simulink model "ben2csys"  (Simulink 6.0)
settings: Solver=ode15s  SolverMode=SingleTasking  StartTime=0.0  StopTime=10  RelTol=1e-3  AbsTol=1e-6
PreLoadFcn:
  | ben2cdat
values from neighbouring files (symbols this model uses):
  a1 = 0.08197    [ben2adat.m]    (also in ben2bdat.m; ben2cdat.m)
  a10 = 0.4078    [ben2adat.m]    (also in ben2bdat.m; ben2cdat.m)
  a11 = 0.3077    [ben2adat.m]    (also in ben2bdat.m; ben2cdat.m)
  a12 = 3.2314    [ben2adat.m]    (also in ben2bdat.m; ben2cdat.m)
  a13 = 0.8597    [ben2adat.m]    (also in ben2bdat.m; ben2cdat.m)
  a14 = -0.002323    [ben2adat.m]    (also in ben2bdat.m; ben2cdat.m)
  a15 = -0.01139    [ben2adat.m]    (also in ben2bdat.m; ben2cdat.m)
  a16 = 45.112    [ben2adat.m]    (also in ben2bdat.m; ben2cdat.m)
  a2 = 0.02296    [ben2adat.m]    (also in ben2bdat.m; ben2cdat.m)
  a3 = -0.004879    [ben2adat.m]    (also in ben2bdat.m; ben2cdat.m)
  a4 = -0.03402    [ben2adat.m]    (also in ben2bdat.m; ben2cdat.m)
  a5 = 0.2551    [ben2adat.m]    (also in ben2bdat.m; ben2cdat.m)
  a6 = 0.02549    [ben2adat.m]    (also in ben2bdat.m; ben2cdat.m)
  a7 = -0.1199    [ben2adat.m]    (also in ben2bdat.m; ben2cdat.m)
  a8 = -0.4283    [ben2adat.m]    (also in ben2bdat.m; ben2cdat.m)
  a9 = 0.6645    [ben2adat.m]    (also in ben2bdat.m; ben2cdat.m)
  b1 = 0.007429    [ben2adat.m]    (also in ben2bdat.m; ben2cdat.m)
  b10 = -0.1037    [ben2adat.m]    (also in ben2bdat.m; ben2cdat.m)
  b11 = 0.3077    [ben2adat.m]    (also in ben2bdat.m; ben2cdat.m)
  b12 = 3.2314    [ben2adat.m]    (also in ben2bdat.m; ben2cdat.m)
  b13 = 0    [ben2adat.m]    (also in ben2bdat.m; ben2cdat.m)
  b14 = 0.002115    [ben2adat.m]    (also in ben2bdat.m; ben2cdat.m)
  b15 = -0.01139    [ben2adat.m]    (also in ben2bdat.m; ben2cdat.m)
  b16 = 45.112    [ben2adat.m]    (also in ben2bdat.m; ben2cdat.m)
  b17 = 0.4040    (= 0.404)    [ben2adat.m]    (also in ben2bdat.m; ben2cdat.m)
  b2 = 0.0752    [ben2adat.m]    (also in ben2bdat.m; ben2cdat.m)
  b3 = 0.06919    [ben2adat.m]    (also in ben2bdat.m; ben2cdat.m)
  b4 = -0.8272    [ben2adat.m]    (also in ben2bdat.m; ben2cdat.m)
  b5 = 0.03861    [ben2adat.m]    (also in ben2bdat.m; ben2cdat.m)
  b6 = -0.3616    [ben2adat.m]    (also in ben2bdat.m; ben2cdat.m)
  b7 = -0.3930    (= -0.393)    [ben2adat.m]    (also in ben2bdat.m; ben2cdat.m)
  b8 = -0.03882    [ben2adat.m]    (also in ben2bdat.m; ben2cdat.m)
  b9 = 0.8064    [ben2adat.m]    (also in ben2bdat.m; ben2cdat.m)
  c1 = -0.01523    [ben2adat.m]    (also in ben2bdat.m; ben2cdat.m)
  c2 = 0.06768    [ben2adat.m]    (also in ben2bdat.m; ben2cdat.m)
  c3 = 0.01514    [ben2adat.m]    (also in ben2bdat.m; ben2cdat.m)
  c4 = 0.002194    [ben2adat.m]    (also in ben2bdat.m; ben2cdat.m)
  c5 = 0.07528    [ben2adat.m]    (also in ben2bdat.m; ben2cdat.m)
  c6 = 0.0002996    [ben2adat.m]    (also in ben2bdat.m = -0.0002996; ben2cdat.m = -0.0002996)
  c7 = 3030.76    [ben2adat.m]    (also in ben2bdat.m; ben2cdat.m)
  gd1 = 1    [ben2adat.m]    (also in ben2bdat.m; ben2cdat.m = [1/950,1]; ben3adat.m = [1,6,13]; ben3bdat.m = [1,6,13])
  gd10 = [1/28,1.4536,1]    [ben2adat.m]    (also in ben2bdat.m; ben2cdat.m)
  gd11 = k13    (= 2.9)    [ben2adat.m]    (also in ben2bdat.m; ben2cdat.m)
  gd12 = [1/325/325,0.5/325,1]    [ben2adat.m]    (also in ben2bdat.m; ben2cdat.m; ben3bdat.m = [1,0])
  gd131 = [1/665/665,.8/665,1]    [ben2cdat.m]    (also in ben3bdat.m = [T2,0])
  gd132 = [1/260/260,0.5/260,1]    [ben2cdat.m]    (also in ben3bdat.m = [1,-1.785,.9988])
  gd13d = [1/2500,1]    [ben2cdat.m]
  gd14 = 1    [ben2adat.m]    (also in ben2bdat.m; ben2cdat.m)
  gd15 = [1,0]    [ben2adat.m]    (also in ben2bdat.m; ben2cdat.m)
  gd161 = [1/70,1]    [ben2bdat.m]    (also in ben2cdat.m)
  gd162 = [1/165/165,1/165,1]    [ben2bdat.m]    (also in ben2cdat.m)
  gd163 = [1/725/725,.8/725,1]    [ben2cdat.m]
  gd17 = [1,0]    [ben2adat.m]    (also in ben2bdat.m; ben2cdat.m)
  gd2 = [1/220,1]    [ben2adat.m]    (also in ben2bdat.m; ben2cdat.m; ben3adat.m = [1,6,13]; ben3bdat.m = [1,6,13])
  gd3 = [1/85/85,1.2/85,1]    [ben2adat.m]    (also in ben2bdat.m; ben2cdat.m; ben3adat.m = [1,-1]; ben3bdat.m = [1,-1])
  gd4 = 1    [ben2adat.m]    (also in ben2bdat.m; ben2cdat.m = [1/775/775,1/775,1]; ben3adat.m = [1,-0.6667]; ben3bdat.m = [1,-0.6667])
  gd5 = [1/170,1]    [ben2adat.m]    (also in ben2bdat.m; ben2cdat.m; ben3adat.m = [1,-1]; ben3bdat.m = [1,-1])
  gd61 = [1/80,1]    [ben2adat.m]    (also in ben2bdat.m; ben2cdat.m)
  gd62 = [1/160/160,0.6/160,1]    [ben2adat.m]    (also in ben2bdat.m; ben2cdat.m)
  gd63 = [1/1600,1]    [ben2adat.m]    (also in ben2bdat.m; ben2cdat.m)
  gd64 = [1/250/250,.6/250,1]    [ben2cdat.m]
  gd65 = [1/300/300,.6/300,1]    [ben2cdat.m]
  gd66 = [1/575/575,.8/575,1]    [ben2cdat.m]
  gd67 = [1/500/500,.6/500,1]    [ben2cdat.m]
  gd7 = [1,0]    [ben2adat.m]    (also in ben2bdat.m; ben2cdat.m; ben3adat.m = [1,-0.9277]; ben3bdat.m = [1,-0.9277])
  gd8 = 1    [ben2adat.m]    (also in ben2bdat.m; ben2cdat.m = [1/526.3,1])
  gd91 = [1,0]    [ben2adat.m]    (also in ben2bdat.m; ben2cdat.m; ben3bdat.m = [1,.25*200,200*200])
  gd92 = [1/50,1]    [ben2adat.m]    (also in ben2bdat.m; ben2cdat.m; ben3bdat.m = [1,0])
  gn1 = 1    [ben2adat.m]    (also in ben2bdat.m; ben2cdat.m; ben3adat.m = -15*[1,1.5]; ben3bdat.m = -15*[1,1.5])
  gn10 = [-1,0]    [ben2adat.m]    (also in ben2bdat.m; ben2cdat.m)
  gn11 = k14    (= 0.66)    [ben2adat.m]    (also in ben2bdat.m; ben2cdat.m)
  gn12 = [1,0]    [ben2adat.m]    (also in ben2bdat.m; ben2cdat.m; ben3bdat.m = 1)
  gn131 = [1/665/665,.08/665,1]    [ben2cdat.m]    (also in ben3bdat.m = [1,-1])
  gn132 = [1/800/800,.12/800,1]    [ben2cdat.m]    (also in ben3bdat.m = .9994*[1,-1.786,1])
  gn13d = [0.4/130,0.4]    [ben2cdat.m]
  gn14 = 0.2 * k14    (= 0.132)    [ben2adat.m]    (also in ben2bdat.m; ben2cdat.m)
  gn15 = [1/30,1]    [ben2adat.m]    (also in ben2bdat.m; ben2cdat.m)
  gn161 = [1/45,1]    [ben2bdat.m]    (also in ben2cdat.m)
  gn162 = 1    [ben2bdat.m]    (also in ben2cdat.m)
  gn163 = [1/725/725,.08/725,1]    [ben2cdat.m]
  gn17 = k12    (= 0.565)    [ben2adat.m]    (also in ben2bdat.m; ben2cdat.m)
  gn2 = 1    [ben2adat.m]    (also in ben2bdat.m; ben2cdat.m; ben3adat.m = [-0.1,9]; ben3bdat.m = [-0.1,9])
  gn3 = 1    [ben2adat.m]    (also in ben2bdat.m; ben2cdat.m; ben3adat.m = .2625*[1,-0.9048]; ben3bdat.m = .2625*[1,-0.9048])
  gn4 = 1    [ben2adat.m]    (also in ben2bdat.m; ben2cdat.m; ben3adat.m = 1.7*[1,-0.9608]; ben3bdat.m = 1.7*[1,-0.9608])
  gn5 = 1    [ben2adat.m]    (also in ben2bdat.m; ben2cdat.m; ben3adat.m = 1.035*[1,-0.9324]; ben3bdat.m = 1.035*[1,-0.9324])
  gn61 = [1,0]    [ben2adat.m]    (also in ben2bdat.m; ben2cdat.m)
  gn62 = [1/30,1]    [ben2adat.m]    (also in ben2bdat.m; ben2cdat.m)
  gn63 = 1    [ben2adat.m]    (also in ben2bdat.m; ben2cdat.m)
  gn64 = [1/250/250,.06/250,1]    [ben2cdat.m]
  gn65 = [1/350/350,.06/350,1]    [ben2cdat.m]
  gn66 = [1/660/660,.4/660,1]    [ben2cdat.m]
  gn67 = [1/850/850,.06/850,1]    [ben2cdat.m]
  gn7 = 1    [ben2adat.m]    (also in ben2bdat.m; ben2cdat.m; ben3adat.m = 0.0362*[1,1]; ben3bdat.m = 0.0362*[1,1])
  gn8 = 1    [ben2adat.m]    (also in ben2bdat.m; ben2cdat.m = [(-1)/526.1,1])
  gn91 = [1,1.5]    [ben2adat.m]    (also in ben2bdat.m; ben2cdat.m; ben3bdat.m = 40000)
  gn92 = [1/150,1]    [ben2adat.m]    (also in ben2bdat.m; ben2cdat.m; ben3bdat.m = 1)
  k1 = 1    [ben2adat.m]    (also in ben2bdat.m; ben2cdat.m)
  k10 = 0    [ben2adat.m]    (also in ben2bdat.m; ben2cdat.m = 0.2)
  k11 = 0.0112    [ben2adat.m]    (also in ben2bdat.m; ben2cdat.m)
  k2 = 1.25    [ben2adat.m]    (also in ben2bdat.m; ben2cdat.m)
  k3 = 0.001244    [ben2adat.m]    (also in ben2bdat.m; ben2cdat.m)
  k4 = 0.1    [ben2adat.m]    (also in ben2bdat.m; ben2cdat.m)
  k5 = 0.01125    [ben2adat.m]    (also in ben2bdat.m; ben2cdat.m)
  k6 = 0.06    [ben2adat.m]    (also in ben2bdat.m; ben2cdat.m)
  k7 = 0    [ben2adat.m]    (also in ben2bdat.m; ben2cdat.m = 0.5)
  k8 = 0    [ben2adat.m]    (also in ben2bdat.m; ben2cdat.m = 0.2)
  k9 = 29.82    [ben2adat.m]    (also in ben2bdat.m; ben2cdat.m)
settings Model: Creator=The MathWorks Inc.  LastModifiedBy=batserve  ExtModeTrigMode=oneshot  ExtModeArmWhenConnect=off  ExtModeAutoUpdateStatusClock=off
settings DataIOCC: ExternalInput=[]  InitialState=[]  LimitDataPoints=off  SaveOutput=off  SaveTime=off
settings OptimizationCC: BooleanDataType=off
settings DebuggingCC: CheckExecutionContextPreStartOutputMsg=on  CheckExecutionContextRuntimeOutputMsg=on  SolverPrmCheckMsg=none  IntegerOverflowMsg=none
settings HardwareCC: TargetUnknown=on

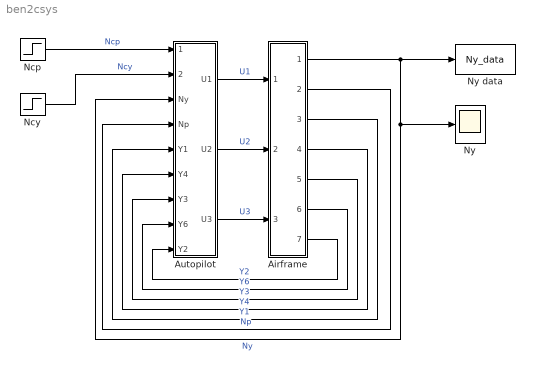
== system ben2csys ==
  Airframe : Subsystem  PropExecContextAcrossSSBoundary=on
  Autopilot : Subsystem  PropExecContextAcrossSSBoundary=on
  Ncp : Step  Time=0  After=0  SampleTime=0
  Ncy : Step  Time=0  SampleTime=0
  Ny : Scope
      settings: TickLabels=on  TimeRange=10  YMin=-0.2  YMax=1.6  DataFormat=Array
  Ny data : ToWorkspace  VariableName=Ny_data  SampleTime=-1  SaveFormat=Array
  wires:
  Airframe/7(Y2) -> Autopilot/9(Y2)  "Y2"
  Airframe/6(Y6) -> Autopilot/8(Y6)  "Y6"
  Airframe/5(Y3) -> Autopilot/7(Y3)  "Y3"
  Airframe/4(Y4) -> Autopilot/6(Y4)  "Y4"
  Airframe/3(Y1) -> Autopilot/5(Y1)  "Y1"
  Airframe/2(Np) -> Autopilot/4(Np)  "Np"
  Ncp/1 -> Autopilot/1(Ncp)  "Ncp"
  Autopilot/1(U1) -> Airframe/1(U1)  "U1"
  Autopilot/2(U2) -> Airframe/2(U2)  "U2"
  Autopilot/3(U3) -> Airframe/3(U3)  "U3"
  Ncy/1 -> Autopilot/2(Ncy)  "Ncy"
  Airframe/1(Ny) -> Ny/1, Autopilot/3(Ny), Ny data/1  "Ny"

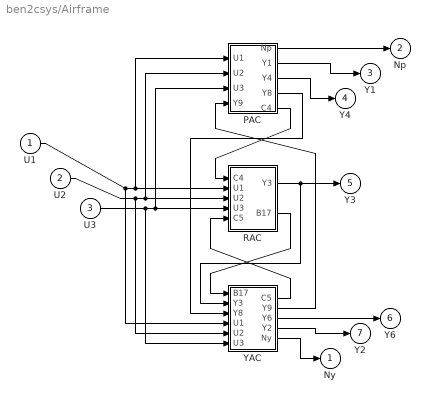
== system ben2csys/Airframe ==
  U1 : Inport  Port=1  LatchInput=off
  U2 : Inport  Port=2  LatchInput=off
  U3 : Inport  Port=3  LatchInput=off
  PAC : Subsystem  PropExecContextAcrossSSBoundary=on
  RAC : Subsystem  PropExecContextAcrossSSBoundary=on
  YAC : Subsystem  PropExecContextAcrossSSBoundary=on
  Ny : Outport  InitialOutput=0
  Np : Outport  Port=2  InitialOutput=0
  Y1 : Outport  Port=3  InitialOutput=0
  Y4 : Outport  Port=4  InitialOutput=0
  Y3 : Outport  Port=5  InitialOutput=0
  Y6 : Outport  Port=6  InitialOutput=0
  Y2 : Outport  Port=7  InitialOutput=0
  wires:
  PAC/5(C4) -> RAC/1(C4)
  PAC/1(Np) -> Np/1
  PAC/2(Y1) -> Y1/1
  PAC/3(Y4) -> Y4/1
  RAC/2(B17) -> YAC/1(B17)
  YAC/5(Ny) -> Ny/1
  YAC/4(Y2) -> Y2/1
  YAC/3(Y6) -> Y6/1
  YAC/2(Y9) -> PAC/4(Y9)
  PAC/4(Y8) -> YAC/3(Y8)
  YAC/1(C5) -> RAC/5(C5)
  RAC/1(Y3) -> Y3/1, YAC/2(Y3)
  U1/1 -> YAC/4(U1), RAC/2(U1), PAC/1(U1)
  U2/1 -> YAC/5(U2), RAC/3(U2), PAC/2(U2)
  U3/1 -> YAC/6(U3), RAC/4(U3), PAC/3(U3)

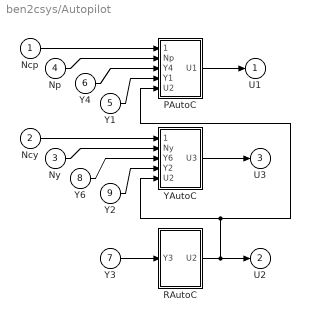
== system ben2csys/Autopilot ==
  Ncp : Inport  Port=1  LatchInput=off
  Ncy : Inport  Port=2  LatchInput=off
  Ny : Inport  Port=3  LatchInput=off
  Np : Inport  Port=4  LatchInput=off
  Y1 : Inport  Port=5  LatchInput=off
  Y4 : Inport  Port=6  LatchInput=off
  Y3 : Inport  Port=7  LatchInput=off
  Y6 : Inport  Port=8  LatchInput=off
  Y2 : Inport  Port=9  LatchInput=off
  PAutoC : Subsystem  PropExecContextAcrossSSBoundary=on
  RAutoC : Subsystem  PropExecContextAcrossSSBoundary=on
  YAutoC : Subsystem  PropExecContextAcrossSSBoundary=on
  U1 : Outport  InitialOutput=0
  U2 : Outport  Port=2  InitialOutput=0
  U3 : Outport  Port=3  InitialOutput=0
  wires:
  RAutoC/1(U2) -> U2/1, YAutoC/5(U2), PAutoC/5(U2)
  Y3/1 -> RAutoC/1(Y3)
  Y2/1 -> YAutoC/4(Y2)
  YAutoC/1(U3) -> U3/1
  Y6/1 -> YAutoC/3(Y6)
  Ny/1 -> YAutoC/2(Ny)
  Ncy/1 -> YAutoC/1(Ncy)
  Y1/1 -> PAutoC/4(Y1)
  PAutoC/1(U1) -> U1/1
  Y4/1 -> PAutoC/3(Y4)
  Np/1 -> PAutoC/2(Np)
  Ncp/1 -> PAutoC/1(Ncp)

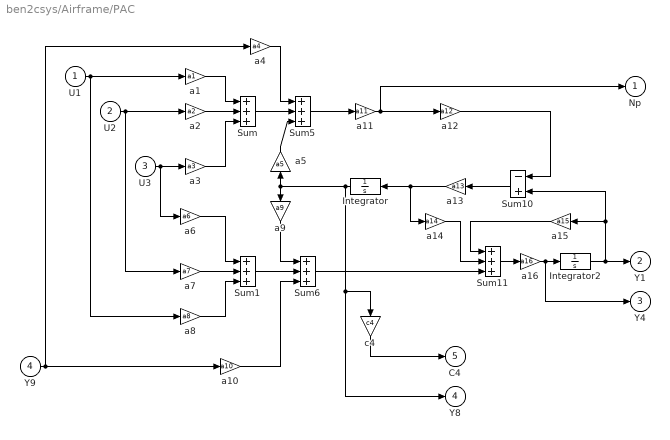
== system ben2csys/Airframe/PAC ==
  U1 : Inport  Port=1  LatchInput=off
  U2 : Inport  Port=2  LatchInput=off
  U3 : Inport  Port=3  LatchInput=off
  Y9 : Inport  Port=4  LatchInput=off
  Integrator : Integrator  Orientation=left
  Integrator2 : Integrator
  Sum{,1,5..6,11} (5 alike) : Sum  Inputs=3  SaturateOnIntegerOverflow=on  InputSameDT=on
  Sum10 : Sum  Orientation=left  Inputs=-+  SaturateOnIntegerOverflow=on  InputSameDT=on
  a1 : Gain  Gain=a1  SaturateOnIntegerOverflow=on
  a10 : Gain  Gain=a10  SaturateOnIntegerOverflow=on
  a11 : Gain  Gain=a11  SaturateOnIntegerOverflow=on
  a12 : Gain  Gain=a12  SaturateOnIntegerOverflow=on
  a13 : Gain  Orientation=left  Gain=a13  SaturateOnIntegerOverflow=on
  a14 : Gain  Gain=a14  SaturateOnIntegerOverflow=on
  a15 : Gain  Orientation=left  Gain=a15  SaturateOnIntegerOverflow=on
  a16 : Gain  Gain=a16  SaturateOnIntegerOverflow=on
  a2 : Gain  Gain=a2  SaturateOnIntegerOverflow=on
  a3 : Gain  Gain=a3  SaturateOnIntegerOverflow=on
  a4 : Gain  Gain=a4  SaturateOnIntegerOverflow=on
  a5 : Gain  Orientation=up  Gain=a5  SaturateOnIntegerOverflow=on
  a6 : Gain  Gain=a6  SaturateOnIntegerOverflow=on
  a7 : Gain  Gain=a7  SaturateOnIntegerOverflow=on
  a8 : Gain  Gain=a8  SaturateOnIntegerOverflow=on
  a9 : Gain  Orientation=down  Gain=a9  SaturateOnIntegerOverflow=on
  c4 : Gain  Orientation=down  Gain=c4  SaturateOnIntegerOverflow=on
  Np : Outport  InitialOutput=0
  Y1 : Outport  Port=2  InitialOutput=0
  Y4 : Outport  Port=3  InitialOutput=0
  Y8 : Outport  Port=4  InitialOutput=0
  C4 : Outport  Port=5  InitialOutput=0
  wires:
  a1/1 -> Sum/1
  a3/1 -> Sum/3
  a8/1 -> Sum1/3
  a6/1 -> Sum1/1
  Integrator2/1 -> Sum10/2, a15/1, Y1/1
  a13/1 -> a14/1, Integrator/1
  Sum/1 -> Sum5/2
  a5/1 -> Sum5/3
  a4/1 -> Sum5/1
  Sum5/1 -> a11/1
  a11/1 -> Np/1, a12/1
  a12/1 -> Sum10/1
  Sum10/1 -> a13/1
  Sum6/1 -> Sum11/3
  a14/1 -> Sum11/2
  a15/1 -> Sum11/1
  Sum11/1 -> a16/1
  a10/1 -> Sum6/3
  Sum1/1 -> Sum6/2
  a9/1 -> Sum6/1
  a16/1 -> Y4/1, Integrator2/1
  U3/1 -> a6/1, a3/1
  a7/1 -> Sum1/2
  a2/1 -> Sum/2
  U1/1 -> a8/1, a1/1
  U2/1 -> a7/1, a2/1
  Y9/1 -> a10/1, a4/1
  Integrator/1 -> c4/1, Y8/1, a9/1, a5/1
  c4/1 -> C4/1

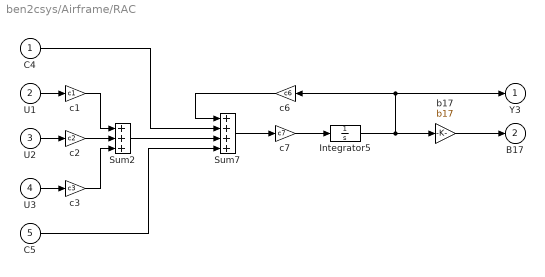
== system ben2csys/Airframe/RAC ==
  C4 : Inport  Port=1  LatchInput=off
  U1 : Inport  Port=2  LatchInput=off
  U2 : Inport  Port=3  LatchInput=off
  U3 : Inport  Port=4  LatchInput=off
  C5 : Inport  Port=5  LatchInput=off
  Integrator5 : Integrator
  Sum2 : Sum  Inputs=3  SaturateOnIntegerOverflow=on  InputSameDT=on
  Sum7 : Sum  Inputs=4  SaturateOnIntegerOverflow=on  InputSameDT=on
  b17 : Gain  Gain=b17  SaturateOnIntegerOverflow=on
  c1 : Gain  Gain=c1  SaturateOnIntegerOverflow=on
  c2 : Gain  Gain=c2  SaturateOnIntegerOverflow=on
  c3 : Gain  Gain=c3  SaturateOnIntegerOverflow=on
  c6 : Gain  Orientation=left  Gain=c6  SaturateOnIntegerOverflow=on
  c7 : Gain  Gain=c7  SaturateOnIntegerOverflow=on
  Y3 : Outport  InitialOutput=0
  B17 : Outport  Port=2  InitialOutput=0
  wires:
  Integrator5/1 -> Y3/1, c6/1, b17/1
  b17/1 -> B17/1
  c6/1 -> Sum7/1
  c7/1 -> Integrator5/1
  Sum7/1 -> c7/1
  C5/1 -> Sum7/4
  C4/1 -> Sum7/2
  Sum2/1 -> Sum7/3
  U3/1 -> c3/1
  c3/1 -> Sum2/3
  c1/1 -> Sum2/1
  U1/1 -> c1/1
  c2/1 -> Sum2/2
  U2/1 -> c2/1

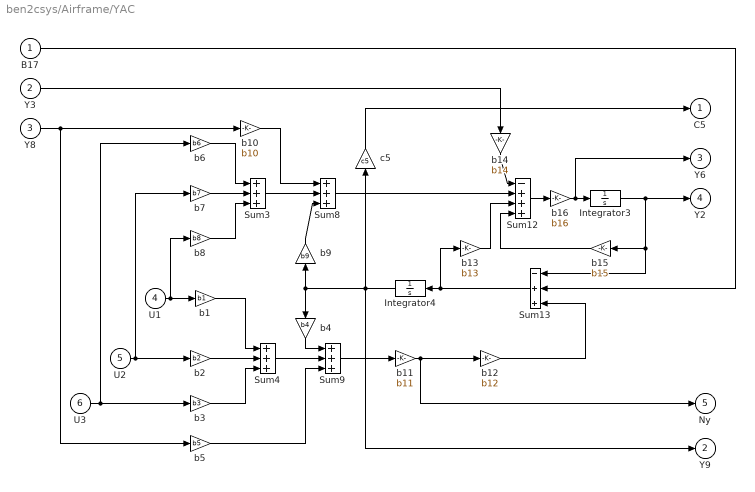
== system ben2csys/Airframe/YAC ==
  B17 : Inport  Port=1  LatchInput=off
  Y3 : Inport  Port=2  LatchInput=off
  Y8 : Inport  Port=3  LatchInput=off
  U1 : Inport  Port=4  LatchInput=off
  U2 : Inport  Port=5  LatchInput=off
  U3 : Inport  Port=6  LatchInput=off
  Integrator3 : Integrator
  Integrator4 : Integrator  Orientation=left
  Sum12 : Sum  Inputs=-+++  SaturateOnIntegerOverflow=on  InputSameDT=on
  Sum13 : Sum  Orientation=left  Inputs=-++  SaturateOnIntegerOverflow=on  InputSameDT=on
  Sum{3..4,8..9} (4 alike) : Sum  Inputs=3  SaturateOnIntegerOverflow=on  InputSameDT=on
  b1 : Gain  Gain=b1  SaturateOnIntegerOverflow=on
  b10 : Gain  Gain=b10  SaturateOnIntegerOverflow=on
  b11 : Gain  Gain=b11  SaturateOnIntegerOverflow=on
  b12 : Gain  Gain=b12  SaturateOnIntegerOverflow=on
  b13 : Gain  Gain=b13  SaturateOnIntegerOverflow=on
  b14 : Gain  Orientation=down  Gain=b14  SaturateOnIntegerOverflow=on
  b15 : Gain  Orientation=left  Gain=b15  SaturateOnIntegerOverflow=on
  b16 : Gain  Gain=b16  SaturateOnIntegerOverflow=on
  b2 : Gain  Gain=b2  SaturateOnIntegerOverflow=on
  b3 : Gain  Gain=b3  SaturateOnIntegerOverflow=on
  b4 : Gain  Orientation=down  Gain=b4  SaturateOnIntegerOverflow=on
  b5 : Gain  Gain=b5  SaturateOnIntegerOverflow=on
  b6 : Gain  Gain=b6  SaturateOnIntegerOverflow=on
  b7 : Gain  Gain=b7  SaturateOnIntegerOverflow=on
  b8 : Gain  Gain=b8  SaturateOnIntegerOverflow=on
  b9 : Gain  Orientation=up  Gain=b9  SaturateOnIntegerOverflow=on
  c5 : Gain  Orientation=up  Gain=c5  SaturateOnIntegerOverflow=on
  C5 : Outport  InitialOutput=0
  Y9 : Outport  Port=2  InitialOutput=0
  Y6 : Outport  Port=3  InitialOutput=0
  Y2 : Outport  Port=4  InitialOutput=0
  Ny : Outport  Port=5  InitialOutput=0
  wires:
  Integrator3/1 -> Sum13/1, b15/1, Y2/1
  Y3/1 -> b14/1
  b6/1 -> Sum3/1
  b8/1 -> Sum3/3
  Y8/1 -> b5/1, b10/1
  b3/1 -> Sum4/3
  b1/1 -> Sum4/1
  Sum13/1 -> b13/1, Integrator4/1
  c5/1 -> C5/1
  U3/1 -> b6/1, b3/1
  U2/1 -> b7/1, b2/1
  U1/1 -> b8/1, b1/1
  b16/1 -> Y6/1, Integrator3/1
  Sum9/1 -> b11/1
  b11/1 -> Ny/1, b12/1
  Sum8/1 -> Sum12/2
  b5/1 -> Sum9/3
  b4/1 -> Sum9/1
  b9/1 -> Sum8/3
  b2/1 -> Sum4/2
  b13/1 -> Sum12/3
  b15/1 -> Sum12/4
  b10/1 -> Sum8/1
  Sum3/1 -> Sum8/2
  b7/1 -> Sum3/2
  b14/1 -> Sum12/1
  Sum12/1 -> b16/1
  b12/1 -> Sum13/3
  Sum4/1 -> Sum9/2
  Integrator4/1 -> b4/1, b9/1, Y9/1, c5/1
  B17/1 -> Sum13/2

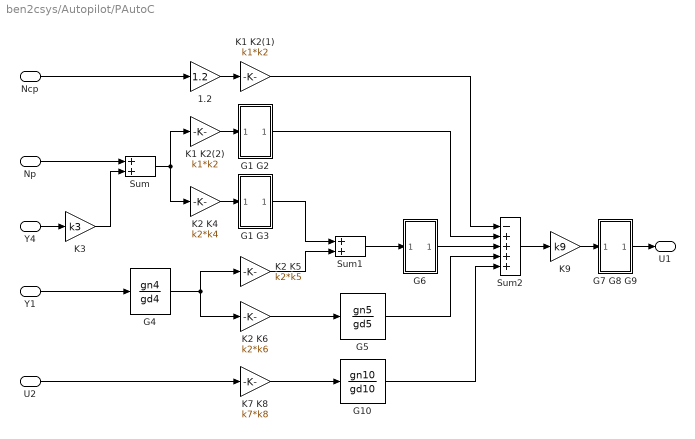
== system ben2csys/Autopilot/PAutoC ==
  Ncp : Inport  Port=1  LatchInput=off
  Np : Inport  Port=2  LatchInput=off
  Y4 : Inport  Port=3  LatchInput=off
  Y1 : Inport  Port=4  LatchInput=off
  U2 : Inport  Port=5  LatchInput=off
  1.2 : Gain  Gain=1.2  SaturateOnIntegerOverflow=on
  G1 G2 : Subsystem  PropExecContextAcrossSSBoundary=on
  G1 G3 : Subsystem  PropExecContextAcrossSSBoundary=on
  G10 : TransferFcn  Numerator=gn10  Denominator=gd10
  G4 : TransferFcn  Numerator=gn4  Denominator=gd4
  G5 : TransferFcn  Numerator=gn5  Denominator=gd5
  G6 : Subsystem  PropExecContextAcrossSSBoundary=on
  G7 G8 G9 : Subsystem  PropExecContextAcrossSSBoundary=on
  K1 K2(1) : Gain  Gain=k1*k2  SaturateOnIntegerOverflow=on
  K1 K2(2) : Gain  Gain=k1*k2  SaturateOnIntegerOverflow=on
  K2 K4 : Gain  Gain=k2*k4  SaturateOnIntegerOverflow=on
  K2 K5 : Gain  Gain=k2*k5  SaturateOnIntegerOverflow=on
  K2 K6 : Gain  Gain=k2*k6  SaturateOnIntegerOverflow=on
  K3 : Gain  Gain=k3  SaturateOnIntegerOverflow=on
  K7 K8 : Gain  Gain=k7*k8  SaturateOnIntegerOverflow=on
  K9 : Gain  Gain=k9  SaturateOnIntegerOverflow=on
  Sum : Sum  Inputs=2  SaturateOnIntegerOverflow=on  InputSameDT=on
  Sum1 : Sum  Inputs=2  SaturateOnIntegerOverflow=on  InputSameDT=on
  Sum2 : Sum  Inputs=-++++  SaturateOnIntegerOverflow=on  InputSameDT=on
  U1 : Outport  InitialOutput=0
  wires:
  G7 G8 G9/1(Out) -> U1/1
  K9/1 -> G7 G8 G9/1(In)
  Y1/1 -> G4/1
  Y4/1 -> K3/1
  Np/1 -> Sum/1
  Ncp/1 -> 1.2/1
  Sum2/1 -> K9/1
  G1 G3/1(Out) -> Sum1/1
  K2 K4/1 -> G1 G3/1(In)
  Sum/1 -> K1 K2(2)/1, K2 K4/1
  K1 K2(2)/1 -> G1 G2/1(In)
  G1 G2/1(Out) -> Sum2/2
  K1 K2(1)/1 -> Sum2/1
  K3/1 -> Sum/2
  G6/1(Out) -> Sum2/3
  Sum1/1 -> G6/1(In)
  G5/1 -> Sum2/4
  K2 K5/1 -> Sum1/2
  1.2/1 -> K1 K2(1)/1
  G4/1 -> K2 K6/1, K2 K5/1
  K2 K6/1 -> G5/1
  U2/1 -> K7 K8/1
  K7 K8/1 -> G10/1
  G10/1 -> Sum2/5

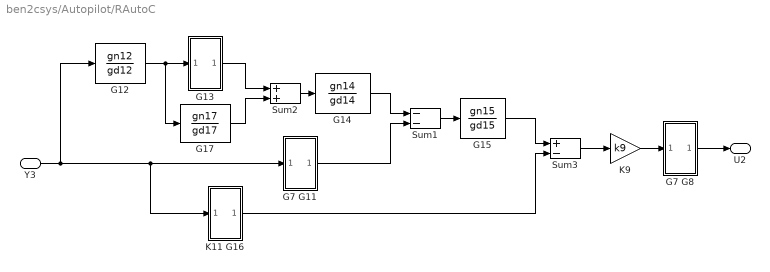
== system ben2csys/Autopilot/RAutoC ==
  Y3 : Inport  Port=1  LatchInput=off
  G12 : TransferFcn  Numerator=gn12  Denominator=gd12
  G13 : Subsystem  PropExecContextAcrossSSBoundary=on
  G14 : TransferFcn  Numerator=gn14  Denominator=gd14
  G15 : TransferFcn  Numerator=gn15  Denominator=gd15
  G17 : TransferFcn  Numerator=gn17  Denominator=gd17
  G7 G11 : Subsystem  PropExecContextAcrossSSBoundary=on
  G7 G8 : Subsystem  PropExecContextAcrossSSBoundary=on
  K11 G16 : Subsystem  PropExecContextAcrossSSBoundary=on
  K9 : Gain  Gain=k9  SaturateOnIntegerOverflow=on
  Sum1 : Sum  Inputs=--  SaturateOnIntegerOverflow=on  InputSameDT=on
  Sum2 : Sum  Inputs=2  SaturateOnIntegerOverflow=on  InputSameDT=on
  Sum3 : Sum  Inputs=+-  SaturateOnIntegerOverflow=on  InputSameDT=on
  U2 : Outport  InitialOutput=0
  wires:
  K11 G16/1(Out) -> Sum3/2
  G15/1 -> Sum3/1
  G7 G11/1(Out) -> Sum1/2
  G12/1 -> G17/1, G13/1(In)
  Sum3/1 -> K9/1
  Sum1/1 -> G15/1
  G14/1 -> Sum1/1
  Sum2/1 -> G14/1
  G13/1(Out) -> Sum2/1
  G17/1 -> Sum2/2
  Y3/1 -> G7 G11/1(In), K11 G16/1(In), G12/1
  G7 G8/1(Out) -> U2/1
  K9/1 -> G7 G8/1(In)

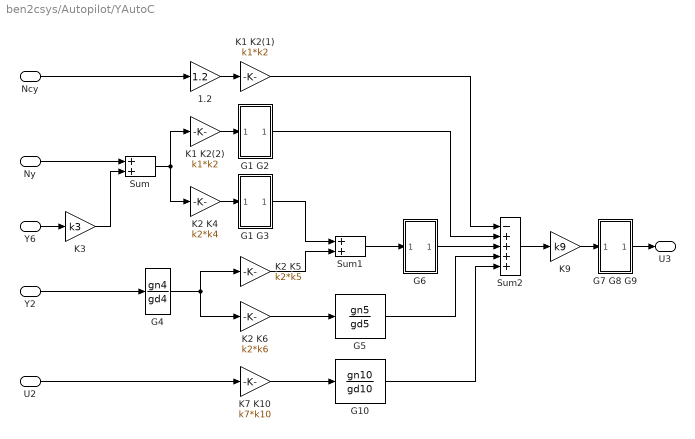
== system ben2csys/Autopilot/YAutoC ==
  Ncy : Inport  Port=1  LatchInput=off
  Ny : Inport  Port=2  LatchInput=off
  Y6 : Inport  Port=3  LatchInput=off
  Y2 : Inport  Port=4  LatchInput=off
  U2 : Inport  Port=5  LatchInput=off
  1.2 : Gain  Gain=1.2  SaturateOnIntegerOverflow=on
  G1 G2 : Subsystem  PropExecContextAcrossSSBoundary=on
  G1 G3 : Subsystem  PropExecContextAcrossSSBoundary=on
  G10 : TransferFcn  Numerator=gn10  Denominator=gd10
  G4 : TransferFcn  Numerator=gn4  Denominator=gd4
  G5 : TransferFcn  Numerator=gn5  Denominator=gd5
  G6 : Subsystem  PropExecContextAcrossSSBoundary=on
  G7 G8 G9 : Subsystem  PropExecContextAcrossSSBoundary=on
  K1 K2(1) : Gain  Gain=k1*k2  SaturateOnIntegerOverflow=on
  K1 K2(2) : Gain  Gain=k1*k2  SaturateOnIntegerOverflow=on
  K2 K4 : Gain  Gain=k2*k4  SaturateOnIntegerOverflow=on
  K2 K5 : Gain  Gain=k2*k5  SaturateOnIntegerOverflow=on
  K2 K6 : Gain  Gain=k2*k6  SaturateOnIntegerOverflow=on
  K3 : Gain  Gain=k3  SaturateOnIntegerOverflow=on
  K7 K10 : Gain  Gain=k7*k10  SaturateOnIntegerOverflow=on
  K9 : Gain  Gain=k9  SaturateOnIntegerOverflow=on
  Sum : Sum  Inputs=2  SaturateOnIntegerOverflow=on  InputSameDT=on
  Sum1 : Sum  Inputs=2  SaturateOnIntegerOverflow=on  InputSameDT=on
  Sum2 : Sum  Inputs=-++++  SaturateOnIntegerOverflow=on  InputSameDT=on
  U3 : Outport  InitialOutput=0
  wires:
  G7 G8 G9/1(Out) -> U3/1
  K9/1 -> G7 G8 G9/1(In)
  Y2/1 -> G4/1
  Y6/1 -> K3/1
  Ny/1 -> Sum/1
  Ncy/1 -> 1.2/1
  Sum2/1 -> K9/1
  G1 G3/1(Out) -> Sum1/1
  K2 K4/1 -> G1 G3/1(In)
  Sum/1 -> K1 K2(2)/1, K2 K4/1
  K1 K2(2)/1 -> G1 G2/1(In)
  G1 G2/1(Out) -> Sum2/2
  K1 K2(1)/1 -> Sum2/1
  K3/1 -> Sum/2
  G6/1(Out) -> Sum2/3
  Sum1/1 -> G6/1(In)
  G5/1 -> Sum2/4
  K2 K5/1 -> Sum1/2
  1.2/1 -> K1 K2(1)/1
  G4/1 -> K2 K6/1, K2 K5/1
  K2 K6/1 -> G5/1
  U2/1 -> K7 K10/1
  K7 K10/1 -> G10/1
  G10/1 -> Sum2/5

== system ben2csys/Autopilot/PAutoC/G1 G2 ==
  In : Inport  Port=1  LatchInput=off
  G1 : TransferFcn  Numerator=gn1  Denominator=gd1
  G2 : TransferFcn  Numerator=gn2  Denominator=gd2
  Out : Outport  InitialOutput=0
  wires:
  G2/1 -> Out/1
  G1/1 -> G2/1
  In/1 -> G1/1

== system ben2csys/Autopilot/PAutoC/G1 G3 ==
  In : Inport  Port=1  LatchInput=off
  G1 : TransferFcn  Numerator=gn1  Denominator=gd1
  G3 : TransferFcn  Numerator=gn3  Denominator=gd3
  Out : Outport  InitialOutput=0
  wires:
  G3/1 -> Out/1
  G1/1 -> G3/1
  In/1 -> G1/1

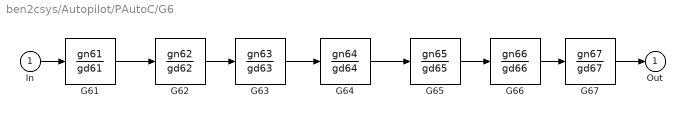
== system ben2csys/Autopilot/PAutoC/G6 ==
  In : Inport  Port=1  LatchInput=off
  G61 : TransferFcn  Numerator=gn61  Denominator=gd61
  G62 : TransferFcn  Numerator=gn62  Denominator=gd62
  G63 : TransferFcn  Numerator=gn63  Denominator=gd63
  G64 : TransferFcn  Numerator=gn64  Denominator=gd64
  G65 : TransferFcn  Numerator=gn65  Denominator=gd65
  G66 : TransferFcn  Numerator=gn66  Denominator=gd66
  G67 : TransferFcn  Numerator=gn67  Denominator=gd67
  Out : Outport  InitialOutput=0
  wires:
  G67/1 -> Out/1
  G66/1 -> G67/1
  G63/1 -> G64/1
  G65/1 -> G66/1
  G64/1 -> G65/1
  In/1 -> G61/1
  G61/1 -> G62/1
  G62/1 -> G63/1

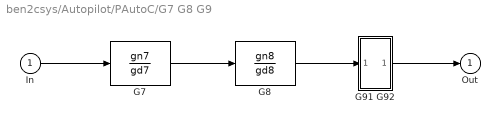
== system ben2csys/Autopilot/PAutoC/G7 G8 G9 ==
  In : Inport  Port=1  LatchInput=off
  G7 : TransferFcn  Numerator=gn7  Denominator=gd7
  G8 : TransferFcn  Numerator=gn8  Denominator=gd8
  G91 G92 : Subsystem  PropExecContextAcrossSSBoundary=on
  Out : Outport  InitialOutput=0
  wires:
  In/1 -> G7/1
  G7/1 -> G8/1
  G8/1 -> G91 G92/1(In)
  G91 G92/1(Out) -> Out/1

== system ben2csys/Autopilot/RAutoC/G13 ==
  In : Inport  Port=1  LatchInput=off
  G131 : TransferFcn  Numerator=gn131  Denominator=gd131
  G132 : TransferFcn  Numerator=gn132  Denominator=gd132
  G13d : TransferFcn  Numerator=gn13d  Denominator=gd13d
  Out : Outport  InitialOutput=0
  wires:
  In/1 -> G13d/1
  G13d/1 -> G131/1
  G131/1 -> G132/1
  G132/1 -> Out/1

== system ben2csys/Autopilot/RAutoC/G7 G11 ==
  In : Inport  Port=1  LatchInput=off
  G11 : TransferFcn  Numerator=gn11  Denominator=gd11
  G7 : TransferFcn  Numerator=gn7  Denominator=gd7
  Out : Outport  InitialOutput=0
  wires:
  G11/1 -> Out/1
  G7/1 -> G11/1
  In/1 -> G7/1

== system ben2csys/Autopilot/RAutoC/G7 G8 ==
  In : Inport  Port=1  LatchInput=off
  G7 : TransferFcn  Numerator=gn7  Denominator=gd7
  G8 : TransferFcn  Numerator=gn8  Denominator=gd8
  Out : Outport  InitialOutput=0
  wires:
  In/1 -> G7/1
  G7/1 -> G8/1
  G8/1 -> Out/1

== system ben2csys/Autopilot/RAutoC/K11 G16 ==
  In : Inport  Port=1  LatchInput=off
  G161 G162 G163 : Subsystem  PropExecContextAcrossSSBoundary=on
  K11 : Gain  Gain=k11  SaturateOnIntegerOverflow=on
  Out : Outport  InitialOutput=0
  wires:
  G161 G162 G163/1(Out) -> Out/1
  K11/1 -> G161 G162 G163/1(In)
  In/1 -> K11/1

== system ben2csys/Autopilot/YAutoC/G1 G2 ==
  In : Inport  Port=1  LatchInput=off
  G1 : TransferFcn  Numerator=gn1  Denominator=gd1
  G2 : TransferFcn  Numerator=gn2  Denominator=gd2
  Out : Outport  InitialOutput=0
  wires:
  G2/1 -> Out/1
  G1/1 -> G2/1
  In/1 -> G1/1

== system ben2csys/Autopilot/YAutoC/G1 G3 ==
  In : Inport  Port=1  LatchInput=off
  G1 : TransferFcn  Numerator=gn1  Denominator=gd1
  G3 : TransferFcn  Numerator=gn3  Denominator=gd3
  Out : Outport  InitialOutput=0
  wires:
  G3/1 -> Out/1
  G1/1 -> G3/1
  In/1 -> G1/1

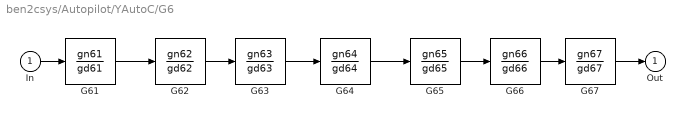
== system ben2csys/Autopilot/YAutoC/G6 ==
  In : Inport  Port=1  LatchInput=off
  G61 : TransferFcn  Numerator=gn61  Denominator=gd61
  G62 : TransferFcn  Numerator=gn62  Denominator=gd62
  G63 : TransferFcn  Numerator=gn63  Denominator=gd63
  G64 : TransferFcn  Numerator=gn64  Denominator=gd64
  G65 : TransferFcn  Numerator=gn65  Denominator=gd65
  G66 : TransferFcn  Numerator=gn66  Denominator=gd66
  G67 : TransferFcn  Numerator=gn67  Denominator=gd67
  Out : Outport  InitialOutput=0
  wires:
  G62/1 -> G63/1
  G61/1 -> G62/1
  In/1 -> G61/1
  G64/1 -> G65/1
  G65/1 -> G66/1
  G63/1 -> G64/1
  G66/1 -> G67/1
  G67/1 -> Out/1

== system ben2csys/Autopilot/YAutoC/G7 G8 G9 ==
  In : Inport  Port=1  LatchInput=off
  G7 : TransferFcn  Numerator=gn7  Denominator=gd7
  G8 : TransferFcn  Numerator=gn8  Denominator=gd8
  G91 G92 : Subsystem  PropExecContextAcrossSSBoundary=on
  Out : Outport  InitialOutput=0
  wires:
  In/1 -> G7/1
  G7/1 -> G8/1
  G8/1 -> G91 G92/1(In)
  G91 G92/1(Out) -> Out/1

== system ben2csys/Autopilot/PAutoC/G7 G8 G9/G91 G92 ==
  In : Inport  Port=1  LatchInput=off
  G91 : TransferFcn  Numerator=gn91  Denominator=gd91
  G92 : TransferFcn  Numerator=gn92  Denominator=gd92
  Out : Outport  InitialOutput=0
  wires:
  G92/1 -> Out/1
  G91/1 -> G92/1
  In/1 -> G91/1

== system ben2csys/Autopilot/RAutoC/K11 G16/G161 G162 G163 ==
  In : Inport  Port=1  LatchInput=off
  G161 : TransferFcn  Numerator=gn161  Denominator=gd161
  G162 : TransferFcn  Numerator=gn162  Denominator=gd162
  G163 : TransferFcn  Numerator=gn163  Denominator=gd163
  Out : Outport  InitialOutput=0
  wires:
  G161/1 -> G162/1
  G162/1 -> G163/1
  In/1 -> G161/1
  G163/1 -> Out/1

== system ben2csys/Autopilot/YAutoC/G7 G8 G9/G91 G92 ==
  In : Inport  Port=1  LatchInput=off
  G91 : TransferFcn  Numerator=gn91  Denominator=gd91
  G92 : TransferFcn  Numerator=gn92  Denominator=gd92
  Out : Outport  InitialOutput=0
  wires:
  G92/1 -> Out/1
  G91/1 -> G92/1
  In/1 -> G91/1
